simulink model "template_Final_Project_MPC5643L"  (Simulink 7.8)
settings: Solver=FixedStepDiscrete  StartTime=0.0  StopTime=10.0  RelTol=1e-3
InitFcn:
  | parameters
values from neighbouring files (symbols this model uses):
  Ak = 100    [parameters.m]
  b = 100    [parameters.m]
  dT = 0.01    [parameters.m]
  H = 10    [parameters.m]
  Kd_PD = 0.04    [parameters.m]
  Kd_PID = 40    [parameters.m]
  Ki_PID = 0    [parameters.m]
  Kp_PD = 0.4    [parameters.m]
  Kp_PID = 500    [parameters.m]
  L1 = 1.6    [parameters.m]
  L2 = 0.8    [parameters.m]
  m = 2000    [parameters.m]
  V_Ki = 50    [parameters.m]
  V_Kp = 5000    [parameters.m]
undefined symbols (not defined in the file or in its folder): A10, A13, A14, A7, A8, AN0, B, B13, B4, B6, B7, B8, C5, C6, D, D11, D4, DiscIntNeverNeededParam, F15, F3, F4, G4, H4, L3, M14, M3, N15, N3, P3, PA10, PA11, PA12, PA13, PA14, PA5, PA6, PA7, PA8, PA9, PB13, PB7, PC11, PC12, PC13, PC14, PC15, PC6, PD0, PD1, PD10, PD11, PD2, PD3, PD4, PD5, PD6, PD7, PD8, PD9, R10 ... (+4)
libraries: Conv_Lib x54, rappid_564xl_ec_toolbox x50, simulink x19, Veh_Sim x9, U_of_M_5643_blockset x1
(part 1 of 2)
settings Model: Creator=lab  LastModifiedBy=jesseku
settings DataIOCC: ExternalInput=off  InitialState=off  SaveOutput=off  SignalLogging=off  SaveTime=off
settings OptimizationCC: InlineParams=on  OptimizeModelRefInitCode=on  LifeSpan=1
settings DebuggingCC: InheritedTsInSrcMsg=none  SingleTaskRateTransMsg=error  UnconnectedInputMsg=error  UnconnectedOutputMsg=error  UnconnectedLineMsg=error  UnknownTsInhSupMsg=error
settings HardwareCC: ProdLargestAtomicInteger=Long  ProdLargestAtomicFloat=Double  ProdIntDivRoundTo=Zero  ProdEndianess=BigEndian  ProdHWDeviceType=Motorola PowerPC
settings RTWCC: SystemTargetFile=rappid564xl.tlc  MakeCommand=rappid_564xl_make_rtw  TemplateMakefile=rappid_564xl_default_tmf  PostCodeGenCommand=rappid_analyzegencode(buildInfo)  Description=RAppID Toolbox MPC564xL Code Generation Target (rappid)  GenerateReport=on  ProcessScript=rappid564xl_make_rtw_hook  IncludeHyperlinkInReport=on  LaunchReport=on
settings CodeAppCC: IgnoreCustomStorageClasses=off
settings STFCustomTargetCC: GeneratePreprocessorConditionals=Use local settings  CombineOutputUpdateFcns=on  SuppressErrorStatus=on  ERTCustomFileBanners=on  SupportContinuousTime=off  SupportNonInlinedSFcns=off  SystemTargetFile=rappid564xl.tlc
settings ERTTargetCC: MultiwordLength=2048  ParMdlRefBuildCompliant=off  CompOptLevelCompliant=off  ConcurrentExecutionCompliant=off  SuppressErrorStatus=on  ERTFirstTimeCompliant=off  ModelStepFunctionPrototypeControlCompliant=off  CPPClassGenCompliant=off  ExtModeMexFile=noextcomm  InlinedParameterPlacement=NonHierarchical  ERTCustomFileTemplate=example_file_process.tlc  ConvertIfToSwitch=off  SuppressUnreachableDefaultCases=off

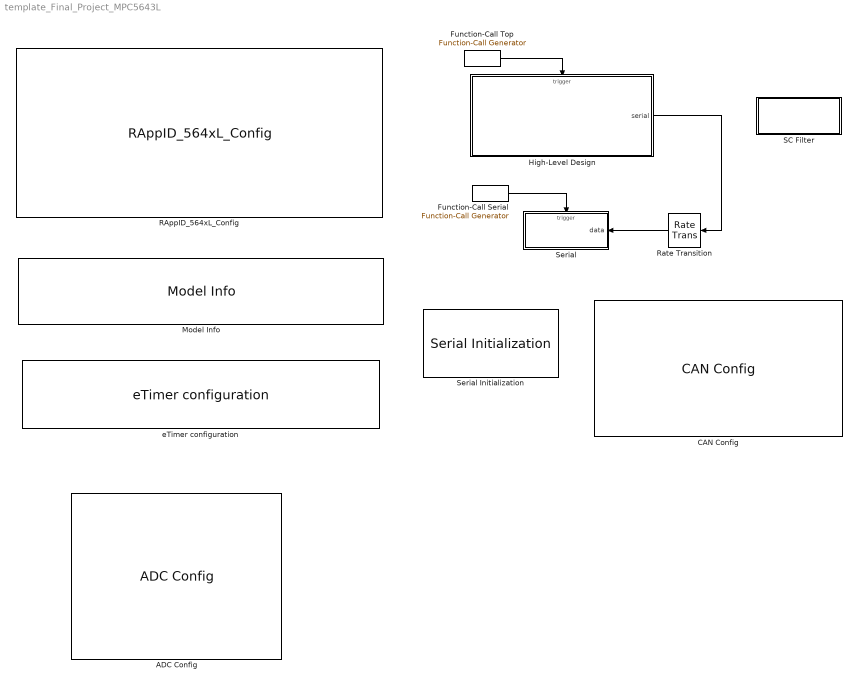
== system template_Final_Project_MPC5643L ==
  ADC Config : rappid_564xl_ec_toolbox/MPC564xL/Motor Control Blocks/ADC Config  adc_unit=0  adc_ctu=off  adc_owr=on  adc_wls=Right  adc_clk=on  adc_ack=on  adc_ctr0_inp=off  adc_ctr0_shft=10 - Avin = 0  adc_ctr0_cmp=01  adc_ctr0_samp=8  adc_ctr1_inp=off  adc_ctr1_cmp=01  adc_ctr1_samp=1  adc_ctr1_tsens=PTAT  adc_pscr_preval=V0  adc_pscr_preconv=off
  CAN Config : rappid_564xl_ec_toolbox/MPC564xL/Communication Blocks/CAN Config  Priority=1  can_unit=A  can_unit_v2=0  can_idam=A - One full ID (standard or extended) per filter element.  can_srx_dis=1 - Self reception disabled  can_presdiv=4  can_rjw=3  can_pseg1=5  can_pseg2=5  can_clk_src=0 - The CAN engine clock source is the oscillator clock  can_lpb=0 - Loop Back disabled  can_smp=0 - One sample is used to determine the bit value  can_boff_rec=0 - Automatic recovering from Bus Off state enabled  can_tsyn=0 - Timer Sync feature disabled  can_lbuf=0 - Buffer with highest priority is transmitted first  can_lom=0 - Listen Only Mode is deactivated  can_propseg=2
  Function-Call Serial : simulink/Ports & Subsystems/Function-Call Generator  sample_time=.05  numberOfIterations=1
  Function-Call Top : simulink/Ports & Subsystems/Function-Call Generator  sample_time=dT  numberOfIterations=1
  High-Level Design : Subsystem
  Model Info : simulink/Model-Wide Utilities/Model Info  InitialBlockCM=None  BlockCM=None  Frame=on  DisplayStringWithTags=|  HorizontalTextAlignment=Center  LeftAlignmentValue=0.5  SourceBlockDiagram=template_Final_Project_MPC5643L  TagMaxNumber=20
      | Model Notes:
      | 
      | You MUST change the CAN IDs whenever you change stations
      | 
      | First 2 buffers must be transmits
  RAppID_564xL_Config : rappid_564xl_ec_toolbox/MPC564xL/RAppID_564xL_Config  SystemClock=120  XTAL=40  MC_clock_60=12  MC_clock_80=16  MC_clock_120=10  SWG_clock_60=20  SWG_clock_80=13.334  SWG_clock_120=20  Compiler=CodeWarrior  MemTarget=FLASH  Part=MPC5643L  Package=144 LQFP  global_int_priority=10  base_tick_priority=11  sys_task_supress=off  exception_handlers=off  stored_mdl_name=adc_pit_block_new  freemaster_interface=Oops  freemaster_rx_pin="LINFlex_0 Rx Pin 116 : \"PB[3]\""  freemaster_tx_pin="LINFlex_0 Tx Pin 114 : \"PB[2]\""  freemaster_interface_1=Serial 0  freemaster_enable=on  freemaster_rate=115200  freemaster_tx0_pin=18 : B[2] : 114 : A14  freemaster_rx0_pin=19 : B[3] : 116 : B13  freemaster_tx1_pin=57 : D[9] : 26 : L3  freemaster_rx1_pin=29 : B[13] : 60 : R10  freemaster_can_channel=1CH  freemater_can_speed=500K  freemaster_can_msgig=0x7AA  ccp_interface=None  ccp_enable=off  ccp_can_channel=CH1 (MB 0 - 1)  ccp_can_speed=500K  ccp_can_cro_id=256  ccp_can_dto_id=257  ccp_dev_id=RappID  ccp_dev_addr=0  ccp_odt=3  ccp_daq=3  pil_enable=off  pil_bam=off  comport=4  pil_rate=115200  bam_password_def=on  bam_password=0xFEEDFACECAFEBEEF  bam_sa_cs=off  bam_start_address=0x0  bam_code_size=0x7000  cons_dspi=on  cons_can=on  cons_adc=on  cons_pwm=on  cons_ctu=on  cons_swg=on  cons_eTimer=on  cons_fm=on
  Rate Transition : RateTransition
  SC Filter : Subsystem
  Serial : Subsystem
  Serial Initialization : U_of_M_5643_blockset/Serial/Serial Initialization
  eTimer configuration : rappid_564xl_ec_toolbox/MPC564xL/Motor Control Blocks/eTimer configuration  SubModule=0  TimerChan=0  subMod=0  channel=0  CountMode=100 - Quadrature count mode using primary and secondary sources  CNTMODE=4  CountOnce=0 - Count repeatedly  ONCE=0  CountLength=0 - Continue counting to roll over  LENGTH=0  CountDirection=0 - Count up  DIR=0  OutputEnable=0 - The external pin is configured as an input  OEN=0  CoChanInit=00 - Other channels cannot force re-initialization of this channel  COINIT=0  StopAction=0 - Output enable is unaffected by stop mode  STPEN=0  ReloadOnCapt=00 - Do not reload the counter on a capture event  ROC=0  PrimarySource=00000 - Counter #0 input pin  PRISRC=0  PrimSrcPol=0 - True polarity  PIPS=0  SecondarySource=00001 - Counter #1 input pin  SECSRC=1  SecSrcPol=0 - True polarity  SIPS=0  FILT_CNT=0  FILT_PER=0  FILT=0  OutputMode=0000 - Software controlled  OUTMODE=0  OutputPol=0 - True polarity  OPS=0  MasterMode=0 - Disable broadcast of this channel output  MSTR=0  ForcedOutVal=0  VAL=0  CoForce=0 - Other channels cannot force this channel output  COFRC=0  CompLoad1=000 - COMP1 is never preload  CLC1=0  CompLoad2=000 - COMP2 is never preload  CLC2=0  CompareMode="00 - COMP1 and COMP2  are used when the counter is counting up"  CMPMODE=0  CaptMode1=00 - Capture disabled  CPT1MODE=0  CaptMode2=00 - Capture disabled  CPT2MODE=0  OneShCaptMode=0 - Free running mode is selected  ONESHOT=0  CaptFIFO=0  CFWM=0  CNTRinit=0  COMP1init=0  COMP2init=0  mod0ch0pin="0   : PA0  : [ 73 ] : [ T14 ]  input/output"  mod0ch1pin="1   : PA1  : [ 74 ] : [ R14 ]  input/output"  mod0ch2pin=None  mod0ch3pin=None  mod0ch4pin=None  mod0ch5pin=None  mod1ch0pin=None  mod1ch1pin=None  mod1ch2pin=None  mod1ch3pin=None  mod1ch4pin=None  mod1ch5pin=None  mod2ch0pin=None  mod2ch1pin=None  mod2ch2pin=None  mod2ch3pin=None  mod2ch4pin=None  mod2ch5pin=None  pcrNum0=0  pcrNum1=1  pcrNum2=255  pcrNum3=255  pcrNum4=255  pcrNum5=255  TCFIE=off  TCF1IE=off  TCF2IE=off  TOFIE=off  IELFIE=off  IEHFIE=off  ICF1IE=off  ICF2IE=off  INTDMA=0
  wires:
  Function-Call Serial/1 -> Serial/Trigger
  Rate Transition/1 -> Serial/1(data)
  Function-Call Top/1 -> High-Level Design/Trigger
  High-Level Design/1(serial) -> Rate Transition/1

== system template_Final_Project_MPC5643L/High-Level Design ==
  Trigger : TriggerPort  TriggerType=function-call
  ACC : Subsystem
  Inputs : Subsystem
  Outputs : Subsystem
  Vehicle_Model : Subsystem
  serial : Outport
  wires:
  Outputs/1(x,y,psi (Cars 1 - 6)) -> serial/1
  Inputs/2(ACC_enable) -> ACC/1(ACC_enable)
  Inputs/1(s,n,psi,us (Cars 1 - 6)) -> ACC/2(s.n.psi,us (Cars 1-6)), Outputs/1(s,n,psi,us (Cars 1 - 6))
  Inputs/3(Cruise Control Speed) -> ACC/3(Cruise Control Speed)
  Inputs/4(Steering Angle (delta)) -> ACC/4(delta)
  Inputs/6(Automatic Steering_enable) -> ACC/6(Automatic Steering_enable)
  ACC/1(Force) -> Vehicle_Model/1(Fd)
  ACC/2(delta (out)) -> Vehicle_Model/2(delta)
  ACC/3(self-aligning torque (out)) -> Vehicle_Model/3(self-align torque (in))
  ACC/4(auto torque (out)) -> Vehicle_Model/4(auto torque (in))
  Vehicle_Model/2(u) -> Outputs/3(u (This Car)), ACC/8(u (in))
  Vehicle_Model/3(self-aligning torque) -> Outputs/4(Self-aligning torque)
  Vehicle_Model/4(auto torque) -> Outputs/5(Auto torque)
  Vehicle_Model/1(s,n,psi,us) -> Outputs/2(s,n,psi,us (This Car)), ACC/7(s.n.psi,us (This Car))
  Inputs/5(Throttle (Fd)) -> ACC/5(Fd)

== system template_Final_Project_MPC5643L/SC Filter ==
  Constant1 : Constant  Value=1e6  OutDataTypeStr=uint32
  Constant2 : Constant  Value=0  OutDataTypeStr=uint32
  Constant3 : Constant  Value=50  OutDataTypeStr=uint32
  Simple PWM Output : rappid_564xl_ec_toolbox/MPC564xL/Motor Control Blocks/Simple PWM Output  Priority=1  pwmModule=0  pwmMod=0  SubModule=1  subMod=1  InitFreq=1000000  resolution=1 %  resValue=1  InitDutyA=0  InitDutyB=50  align=A B - edge aligned  PhaseShift_A=0  PhaseShift=0  Phase_A=0  Phase_B=0  centered=0  DoubleS=off  doubleSw=off  debugSw=off  debug_mode=0  pin_A0=None  pin_B0=None  pin_X0=None  pin_A1=None  pin_B1="38  : PC6  : [ 142 ] : [ D4 ]"  pin_X1=None  pin_A2=None  pin_B2=None  pin_X2=None  pin_A3=None  pin_B3=None  pin_X3=None  pin1_A0=None  pin1_B0=None  pin1_X0=None  pin1_A1=None  pin1_B1=None  pin1_X1=None  pin1_A2=None  pin1_B2=None  pin1_X2=None  pin1_A3=None  pin1_B3=None  pin1_X3=None  pcrNumA=255  pcrNumB=38  pcrNumX=255  polA=off  polB=off  polX=off  octrl=0  syncFrom0=off  masterSync=0  outVal0=off  outVal1=off  outVal2=off  outVal3=off  outVal4=on  outVal5=on  outTrig=48
  wires:
  Constant1/1 -> Simple PWM Output/1
  Constant2/1 -> Simple PWM Output/2
  Constant3/1 -> Simple PWM Output/3

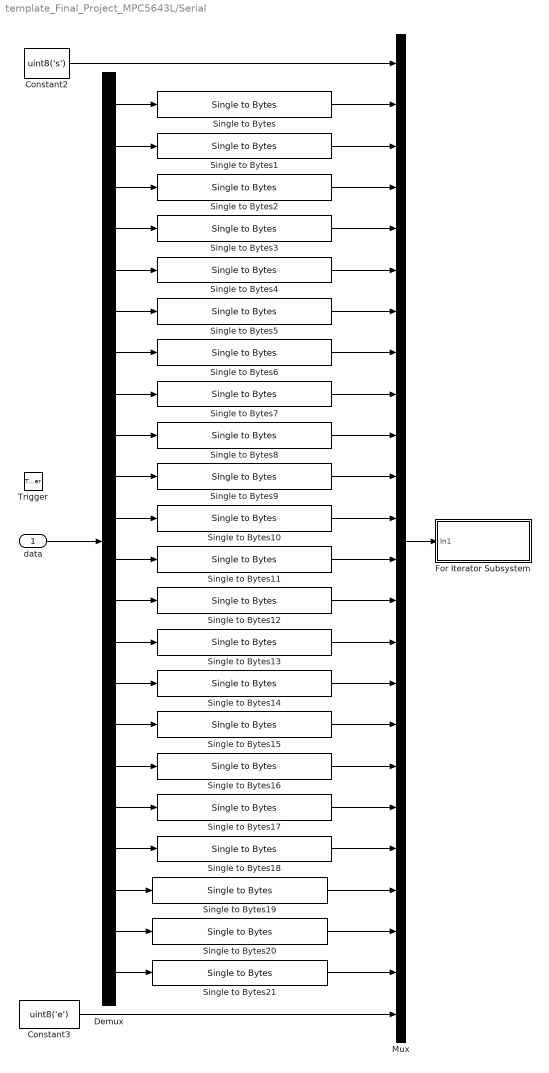
== system template_Final_Project_MPC5643L/Serial ==
  data : Inport
  Trigger : TriggerPort  TriggerType=function-call
  Constant2 : Constant  Value=uint8('s')  OutDataTypeStr=uint8
  Constant3 : Constant  Value=uint8('e')  OutDataTypeStr=uint8
  Demux : Demux  Outputs=22
  For Iterator Subsystem : Subsystem
  Mux : Mux  Inputs=24
  Single to Bytes{,1..21} (22 alike) : Conv_Lib/Single to Bytes
  wires:
  Constant2/1 -> Mux/1
  Single to Bytes/1 -> Mux/2
  Single to Bytes1/1 -> Mux/3
  Single to Bytes2/1 -> Mux/4
  Single to Bytes3/1 -> Mux/5
  Single to Bytes4/1 -> Mux/6
  Single to Bytes5/1 -> Mux/7
  Single to Bytes6/1 -> Mux/8
  Single to Bytes7/1 -> Mux/9
  Single to Bytes8/1 -> Mux/10
  Single to Bytes9/1 -> Mux/11
  Single to Bytes10/1 -> Mux/12
  Single to Bytes11/1 -> Mux/13
  Single to Bytes12/1 -> Mux/14
  Single to Bytes13/1 -> Mux/15
  Single to Bytes15/1 -> Mux/17
  Single to Bytes16/1 -> Mux/18
  Single to Bytes17/1 -> Mux/19
  Mux/1 -> For Iterator Subsystem/1(In1)
  Demux/1 -> Single to Bytes/1
  Demux/2 -> Single to Bytes1/1
  Demux/3 -> Single to Bytes2/1
  Demux/4 -> Single to Bytes3/1
  Demux/5 -> Single to Bytes4/1
  Demux/6 -> Single to Bytes5/1
  Demux/7 -> Single to Bytes6/1
  Demux/8 -> Single to Bytes7/1
  Demux/9 -> Single to Bytes8/1
  Demux/10 -> Single to Bytes9/1
  Demux/11 -> Single to Bytes10/1
  Demux/12 -> Single to Bytes11/1
  Demux/13 -> Single to Bytes12/1
  Demux/14 -> Single to Bytes13/1
  Demux/15 -> Single to Bytes14/1
  Demux/16 -> Single to Bytes15/1
  Demux/17 -> Single to Bytes16/1
  Demux/18 -> Single to Bytes17/1
  data/1 -> Demux/1
  Single to Bytes14/1 -> Mux/16
  Demux/19 -> Single to Bytes18/1
  Demux/20 -> Single to Bytes19/1
  Demux/21 -> Single to Bytes20/1
  Demux/22 -> Single to Bytes21/1
  Single to Bytes18/1 -> Mux/20
  Single to Bytes19/1 -> Mux/21
  Single to Bytes20/1 -> Mux/22
  Single to Bytes21/1 -> Mux/23
  Constant3/1 -> Mux/24

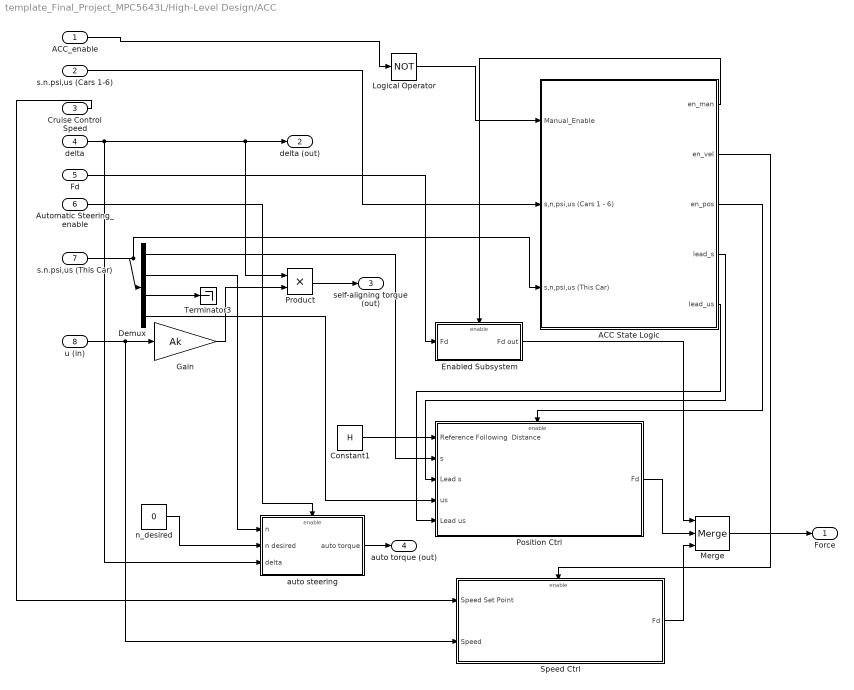
== system template_Final_Project_MPC5643L/High-Level Design/ACC ==
  ACC_enable : Inport
  s.n.psi,us (Cars 1-6) : Inport  Port=2
  Cruise Control Speed : Inport  Port=3
  delta : Inport  Port=4
  Fd : Inport  Port=5
  Automatic Steering_enable : Inport  Port=6
  s.n.psi,us (This Car) : Inport  Port=7
  u (in) : Inport  Port=8
  ACC State Logic : Subsystem
  Constant1 : Constant  Value=H  OutDataTypeStr=single
  Demux : Demux
  Enabled Subsystem : Subsystem  TreatAsAtomicUnit=on
  Gain : Gain  Gain=Ak
  Logical Operator : Logic  Operator=NOT  AllPortsSameDT=off  OutDataTypeStr=boolean
  Merge : Merge  Inputs=3
  Position Ctrl : Subsystem  TreatAsAtomicUnit=on
  Product : Product  OutDataTypeStr=single  RndMeth=Zero
  Speed Ctrl : Subsystem  TreatAsAtomicUnit=on
  Terminator3 : Terminator
  auto steering : Subsystem  TreatAsAtomicUnit=on
  n_desired : Constant  Value=0  OutDataTypeStr=single
  Force : Outport  OutDataTypeStr=single
  delta (out) : Outport  Port=2
  self-aligning torque (out) : Outport  Port=3
  auto torque (out) : Outport  Port=4
  wires:
  ACC_enable/1 -> Logical Operator/1
  delta/1 -> auto steering/3(delta), Product/1, delta (out)/1
  u (in)/1 -> Gain/1, Speed Ctrl/2(Speed)
  Gain/1 -> Product/2
  Product/1 -> self-aligning torque (out)/1
  Logical Operator/1 -> ACC State Logic/1(Manual_Enable)
  s.n.psi,us (Cars 1-6)/1 -> ACC State Logic/2(s,n,psi,us (Cars 1 - 6))
  ACC State Logic/3(en_pos) -> Position Ctrl/Enable
  ACC State Logic/2(en_vel) -> Speed Ctrl/Enable
  ACC State Logic/4(lead_s) -> Position Ctrl/3(Lead s)
  ACC State Logic/5(lead_us) -> Position Ctrl/5(Lead us)
  Cruise Control Speed/1 -> Speed Ctrl/1(Speed Set Point)
  s.n.psi,us (This Car)/1 -> ACC State Logic/3(s,n,psi,us (This Car)), Demux/1
  Demux/1 -> Position Ctrl/2(s)
  Demux/4 -> Position Ctrl/4(us)
  Demux/3 -> Terminator3/1
  Constant1/1 -> Position Ctrl/1(Reference Following  Distance)
  Position Ctrl/1(Fd) -> Merge/2
  Speed Ctrl/1(Fd) -> Merge/3
  Merge/1 -> Force/1
  ACC State Logic/1(en_man) -> Enabled Subsystem/Enable
  Enabled Subsystem/1(Fd out) -> Merge/1
  Fd/1 -> Enabled Subsystem/1(Fd)
  auto steering/1(auto torque) -> auto torque (out)/1
  Demux/2 -> auto steering/1(n)
  n_desired/1 -> auto steering/2(n desired)
  Automatic Steering_enable/1 -> auto steering/Enable

== system template_Final_Project_MPC5643L/High-Level Design/Inputs ==
  ADC Channel : rappid_564xl_ec_toolbox/MPC564xL/Motor Control Blocks/ADC Channel  adc_unit=0  adc_chan0=older  adc_chan0_v2=23 : PB7 : [43] : [R5] : AN0  adc_chan1=older  adc_chan1_v2=29 : PB13 : [60] : [R10] : AN0  simulate=off  interrupt=off  adc_mode=Normal  adc_presample=off
  Data Type Conversion : DataTypeConversion  OutDataTypeStr=single
  Digital Input : rappid_564xl_ec_toolbox/MPC564xL/General Purpose Blocks/Digital Input  gpio_outputs="13  : PA13 : [ 136 ] : [ C6 ]"  pinNum=[ 136 ]  pcrNum=13
  Digital Input1 : rappid_564xl_ec_toolbox/MPC564xL/General Purpose Blocks/Digital Input  gpio_outputs="14  : PA14 : [ 143 ] : [ B4 ]"  pinNum=[ 143 ]  pcrNum=14
  Other Cars : Subsystem
  Scale1 : Subsystem
  Speed_input : Subsystem
  eTimer CNTR Register Read : rappid_564xl_ec_toolbox/MPC564xL/Motor Control Blocks/eTimer CNTR Register Read  SubModule=0  TimerChan=0  subMod=0  channel=0
  s,n,psi,us (Cars 1 - 6) : Outport
  ACC_enable : Outport  Port=2
  Cruise Control Speed : Outport  Port=3
  Steering Angle (delta) : Outport  Port=4
  Throttle (Fd) : Outport  Port=5
  Automatic Steering_enable : Outport  Port=6
  wires:
  Digital Input1/1 -> Automatic Steering_enable/1
  Other Cars/1(s,n,psi,us (Car 1 - 6)) -> s,n,psi,us (Cars 1 - 6)/1
  Digital Input/1 -> ACC_enable/1
  eTimer CNTR Register Read/1 -> Scale1/1(Encoder Counts)
  Scale1/1(Haptic Wheel Position (degrees)) -> Steering Angle (delta)/1
  Speed_input/1(Command Speed) -> Cruise Control Speed/1
  ADC Channel/1 -> Data Type Conversion/1
  Data Type Conversion/1 -> Throttle (Fd)/1

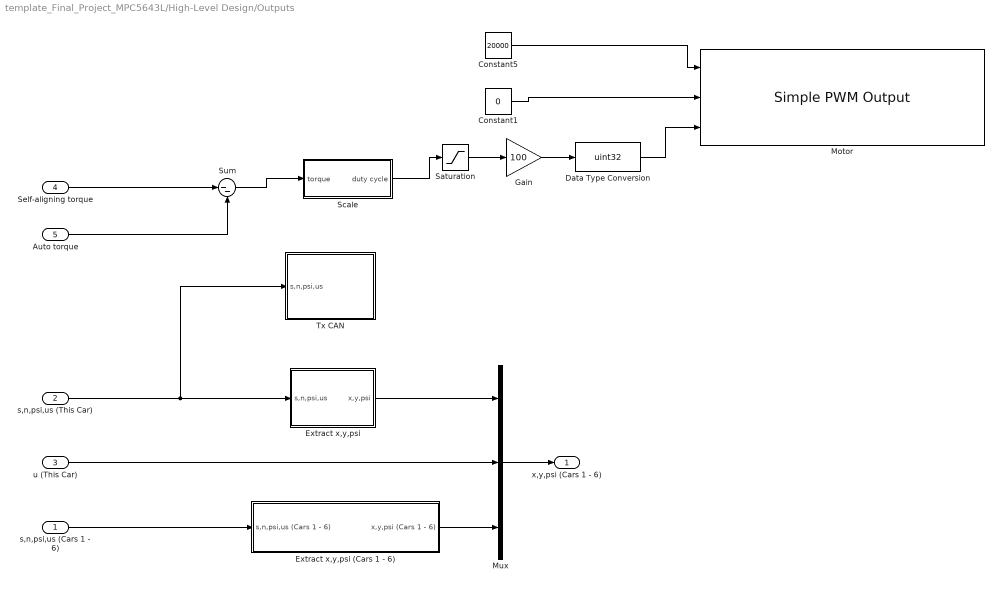
== system template_Final_Project_MPC5643L/High-Level Design/Outputs ==
  s,n,psi,us (Cars 1 - 6) : Inport
  s,n,psi,us (This Car) : Inport  Port=2
  u (This Car) : Inport  Port=3
  Self-aligning torque : Inport  Port=4
  Auto torque : Inport  Port=5
  Constant1 : Constant  Value=0  OutDataTypeStr=uint32
  Constant5 : Constant  Value=20000  OutDataTypeStr=uint32
  Data Type Conversion : DataTypeConversion  OutDataTypeStr=uint32
  Extract x,y,psi : Subsystem
  Extract x,y,psi (Cars 1 - 6) : Subsystem
  Gain : Gain  Gain=100
  Motor : rappid_564xl_ec_toolbox/MPC564xL/Motor Control Blocks/Simple PWM Output  Priority=1  pwmModule=0  pwmMod=0  SubModule=0  subMod=0  InitFreq=20000  resolution=1 %  resValue=1  InitDutyA=0  InitDutyB=0  align=A B - edge aligned  PhaseShift_A=0  PhaseShift=0  Phase_A=0  Phase_B=0  centered=0  DoubleS=off  doubleSw=off  debugSw=off  debug_mode=0  pin_A0=None  pin_B0="59  : PD11 : [ 78 ] : [ R16 ]"  pin_X0=None  pin_A1=None  pin_B1=None  pin_X1=None  pin_A2=None  pin_B2=None  pin_X2=None  pin_A3=None  pin_B3=None  pin_X3=None  pin1_A0=None  pin1_B0=None  pin1_X0=None  pin1_A1=None  pin1_B1=None  pin1_X1=None  pin1_A2=None  pin1_B2=None  pin1_X2=None  pin1_A3=None  pin1_B3=None  pin1_X3=None  pcrNumA=255  pcrNumB=59  pcrNumX=255  polA=off  polB=off  polX=off  octrl=0  syncFrom0=off  masterSync=0  outVal0=off  outVal1=off  outVal2=on  outVal3=on  outVal4=on  outVal5=on  outTrig=60
  Mux : Mux  Inputs=3
  Saturation : Saturate  UpperLimit=.76  LowerLimit=.24
  Scale : Subsystem
  Sum : Sum  Inputs=|--
  Tx CAN : Subsystem
  x,y,psi (Cars 1 - 6) : Outport
  wires:
  s,n,psi,us (Cars 1 - 6)/1 -> Extract x,y,psi (Cars 1 - 6)/1(s,n,psi,us (Cars 1 - 6))
  s,n,psi,us (This Car)/1 -> Extract x,y,psi/1(s,n,psi,us), Tx CAN/1(s,n,psi,us)
  Extract x,y,psi/1(x,y,psi) -> Mux/1
  Mux/1 -> x,y,psi (Cars 1 - 6)/1
  u (This Car)/1 -> Mux/2
  Extract x,y,psi (Cars 1 - 6)/1(x,y,psi (Cars 1 - 6)) -> Mux/3
  Constant1/1 -> Motor/2
  Constant5/1 -> Motor/1
  Saturation/1 -> Gain/1
  Scale/1(duty cycle) -> Saturation/1
  Gain/1 -> Data Type Conversion/1
  Data Type Conversion/1 -> Motor/3
  Sum/1 -> Scale/1(torque)
  Self-aligning torque/1 -> Sum/1
  Auto torque/1 -> Sum/2

== system template_Final_Project_MPC5643L/High-Level Design/Vehicle_Model ==
  Fd : Inport  OutDataTypeStr=single
  delta : Inport  Port=2  OutDataTypeStr=single
  self-align torque (in) : Inport  Port=3
  auto torque (in) : Inport  Port=4
  DTC1 : DataTypeConversion  OutDataTypeStr=single
  DTC2 : DataTypeConversion  OutDataTypeStr=single
  Mux : Mux
  Subsystem : Subsystem
  u to us : Subsystem
  x,y to s,n : Veh_Sim/x,y to s,n  SystemSampleTime=-1
  s,n,psi,us : Outport
  u : Outport  Port=2
  self-aligning torque : Outport  Port=3
  auto torque : Outport  Port=4
  wires:
  Fd/1 -> DTC1/1
  delta/1 -> DTC2/1
  DTC1/1 -> Subsystem/1(Fd)  "Fd"
  DTC2/1 -> u to us/3(delta), Subsystem/2(delta)  "delta"
  self-align torque (in)/1 -> self-aligning torque/1
  auto torque (in)/1 -> auto torque/1
  Subsystem/1(x) -> x,y to s,n/1
  Subsystem/2(y) -> x,y to s,n/2
  Subsystem/4(u) -> u/1, u to us/4(u)
  Subsystem/3(psi) -> u to us/2(psi), Mux/3
  x,y to s,n/1 -> u to us/1(s), Mux/1
  x,y to s,n/2 -> Mux/2
  Mux/1 -> s,n,psi,us/1
  u to us/1(us) -> Mux/4

== system template_Final_Project_MPC5643L/Serial/For Iterator Subsystem ==
  In1 : Inport
  Data Type Conversion : DataTypeConversion  OutDataTypeStr=uint8
  For Iterator : ForIterator  IterationLimit=91  IndexMode=Zero-based  IterationVariableDataType=int8
  Index Vector : MultiPortSwitch  DataPortOrder=Zero-based contiguous  Inputs=1  zeroidx=on
  S-Function : S-Function  FunctionName=SerialSend  EnableBusSupport=off
      mask Display:
      | patch([0 0 1 1], [0 1 1 0], [255/255 255/255 0])
      | patch([0 0 0.05 0.05], [0 1 1 0], [0 0 255/255])
      | patch([1 1 0.95 0.95], [0 1 1 0], [0 0 255/255])
      | 
      | text (0.52, 0.8, ['Serial Send'], 'horizontalAlignment', 'center');
      | %text (0.5, .5, ['System Clock MHz: ' get_param(gcb,'SystemClock')], 'horizontalAlignment', 'center');
      | %text (0.5, .35, ['Baud Rate: ' get_param(gcb,'BaudRate')], 'horizontalAlignment', 'center');
      | text(0.5, 0.1, 'The University of Michigan', 'horizontalAlignment', 'center');
  wires:
  In1/1 -> Index Vector/2
  Index Vector/1 -> Data Type Conversion/1
  For Iterator/1 -> Index Vector/1
  Data Type Conversion/1 -> S-Function/1

== system template_Final_Project_MPC5643L/High-Level Design/ACC/ACC State Logic ==
  Manual_Enable : Inport
  s,n,psi,us (Cars 1 - 6) : Inport  Port=2
  s,n,psi,us (This Car) : Inport  Port=3
  Chart : Stateflow chart  TreatAsAtomicUnit=on
  Constant : Constant  Value=H  OutDataTypeStr=single
  Demux1 : Demux
  Pick_Lead : Subsystem
  Terminator : Terminator
  Terminator16 : Terminator
  Terminator17 : Terminator
  en_man : Outport
  en_vel : Outport  Port=2
  en_pos : Outport  Port=3
  lead_s : Outport  Port=4
  lead_us : Outport  Port=5
  wires:
  Demux1/1 -> Pick_Lead/3(s), Chart/5(s)
  Demux1/2 -> Terminator16/1
  Demux1/3 -> Terminator17/1
  Demux1/4 -> Chart/4(us)
  s,n,psi,us (Cars 1 - 6)/1 -> Pick_Lead/2(si)
  Constant/1 -> Pick_Lead/1(H), Chart/6(H)
  s,n,psi,us (This Car)/1 -> Demux1/1
  Pick_Lead/1(lead_s) -> lead_s/1, Chart/3(si)
  Pick_Lead/2(lead_u) -> lead_us/1, Chart/2(usi)
  Manual_Enable/1 -> Chart/1(enable)
  Chart/1(speed_en) -> en_vel/1
  Chart/2(pos_en) -> en_pos/1
  Chart/3(man_en) -> en_man/1
  Chart/4(state) -> Terminator/1

== system template_Final_Project_MPC5643L/High-Level Design/ACC/Enabled Subsystem ==
  Fd : Inport  OutDataTypeStr=single
  Enable : EnablePort
  Fd out : Outport  OutDataTypeStr=single
  wires:
  Fd/1 -> Fd out/1

== system template_Final_Project_MPC5643L/High-Level Design/ACC/Position Ctrl ==
  note: u
  Reference Following  Distance : Inport
  s : Inport  Port=2
  Lead s : Inport  Port=3
  us : Inport  Port=4
  Lead us : Inport  Port=5
  Enable : EnablePort
  D-gain : Gain  Gain=2.45*m  SaturateOnIntegerOverflow=on  OutDataTypeStr=Inherit: Same as input  ParamDataTypeStr=Inherit: Same as input
  Feed-forward : Gain  Gain=b  SaturateOnIntegerOverflow=on  OutDataTypeStr=Inherit: Same as input  ParamDataTypeStr=Inherit: Same as input
  P-gain : Gain  Gain=-1.5*m  SaturateOnIntegerOverflow=on  OutDataTypeStr=Inherit: Same as input  ParamDataTypeStr=Inherit: Same as input
  Sum1 : Sum  Inputs=|++  SaturateOnIntegerOverflow=on
  Sum2 : Sum  Inputs=+-|  SaturateOnIntegerOverflow=on
  Sum3 : Sum  Inputs=|+-  SaturateOnIntegerOverflow=on
  Sum4 : Sum  Inputs=|+-  SaturateOnIntegerOverflow=on
  Sum5 : Sum  Inputs=|++  SaturateOnIntegerOverflow=on
  Fd : Outport
  wires:
  Lead s/1 -> Sum3/1
  s/1 -> Sum3/2
  Reference Following  Distance/1 -> Sum2/1  "desired distance"
  Sum3/1 -> Sum2/2  "head-way"
  Sum2/1 -> P-gain/1
  P-gain/1 -> Sum1/1
  D-gain/1 -> Sum1/2
  us/1 -> Sum4/2
  Lead us/1 -> Sum4/1, Feed-forward/1
  Sum4/1 -> D-gain/1
  Feed-forward/1 -> Sum5/2
  Sum1/1 -> Sum5/1
  Sum5/1 -> Fd/1  "F"

== system template_Final_Project_MPC5643L/High-Level Design/ACC/Speed Ctrl ==
  Speed Set Point : Inport
  Speed : Inport  Port=2
  Enable : EnablePort
  Gain : Gain  Gain=b  SaturateOnIntegerOverflow=on  OutDataTypeStr=Inherit: Same as input  ParamDataTypeStr=Inherit: Same as input
  PI : Subsystem
  Sum : Sum  Inputs=++|  SaturateOnIntegerOverflow=on
  Sum1 : Sum  Inputs=|+-  SaturateOnIntegerOverflow=on
  Fd : Outport
  wires:
  Speed Set Point/1 -> Gain/1, Sum1/1  "desired speed"
  Speed/1 -> Sum1/2
  Sum1/1 -> PI/1(Error)
  Gain/1 -> Sum/1
  PI/1(U) -> Sum/2
  Sum/1 -> Fd/1  "Fd"

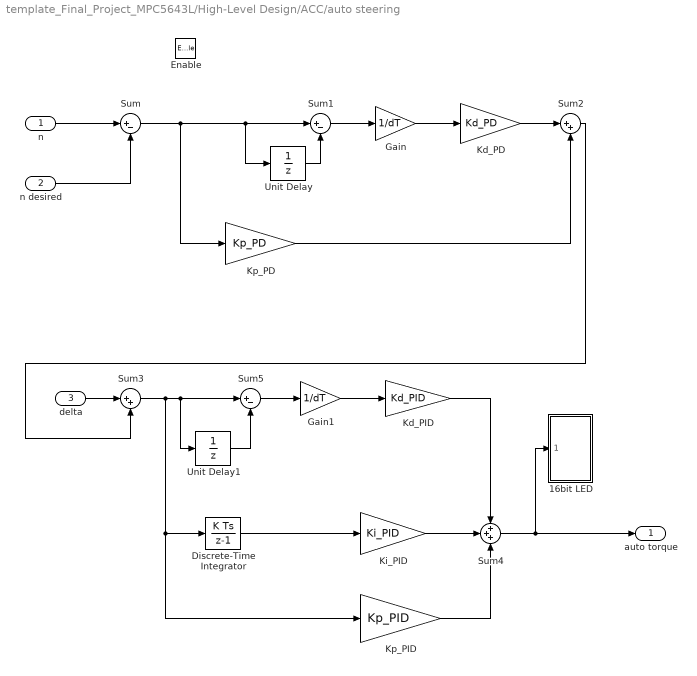
== system template_Final_Project_MPC5643L/High-Level Design/ACC/auto steering ==
  n : Inport
  n desired : Inport  Port=2
  delta : Inport  Port=3
  Enable : EnablePort
  16bit LED : Subsystem
  Discrete-Time Integrator : DiscreteIntegrator  SampleTime=-1  ICPrevOutput=DiscIntNeverNeededParam  ICPrevScaledInput=DiscIntNeverNeededParam
  Gain : Gain  Gain=1/dT
  Gain1 : Gain  Gain=1/dT
  Kd_PD : Gain  Gain=Kd_PD
  Kd_PID : Gain  Gain=Kd_PID
  Ki_PID : Gain  Gain=Ki_PID
  Kp_PD : Gain  Gain=Kp_PD
  Kp_PID : Gain  Gain=Kp_PID
  Sum : Sum  Inputs=|+-
  Sum1 : Sum  Inputs=|+-
  Sum2 : Sum  Inputs=|++
  Sum3 : Sum  Inputs=|++
  Sum4 : Sum  Inputs=+++
  Sum5 : Sum  Inputs=|+-
  Unit Delay : UnitDelay  SampleTime=-1
  Unit Delay1 : UnitDelay  SampleTime=-1
  auto torque : Outport
  wires:
  n/1 -> Sum/1
  n desired/1 -> Sum/2
  Sum/1 -> Sum1/1, Unit Delay/1, Kp_PD/1
  Unit Delay/1 -> Sum1/2
  Sum1/1 -> Gain/1
  Gain/1 -> Kd_PD/1
  Kd_PD/1 -> Sum2/1
  Kp_PD/1 -> Sum2/2
  delta/1 -> Sum3/1
  Kd_PID/1 -> Sum4/1
  Ki_PID/1 -> Sum4/2
  Kp_PID/1 -> Sum4/3
  Discrete-Time Integrator/1 -> Ki_PID/1
  Sum3/1 -> Kp_PID/1, Discrete-Time Integrator/1, Sum5/1, Unit Delay1/1
  Gain1/1 -> Kd_PID/1
  Sum5/1 -> Gain1/1
  Unit Delay1/1 -> Sum5/2
  Sum4/1 -> 16bit LED/1(16 bits), auto torque/1
  Sum2/1 -> Sum3/2

== system template_Final_Project_MPC5643L/High-Level Design/Inputs/Other Cars ==
  "1 for GSI vehicle only, 0 for ALL student vehicles" : Constant  Value=0
  Car1 : Subsystem
  Car2 : Subsystem
  Car3 : Subsystem
  Car4 : Subsystem
  Car5 : Subsystem
  Car6 : Subsystem
  GSI Car : Subsystem
  Mux1 : Mux  Inputs=2
  Mux2 : Mux  Inputs=6
  Switch : Switch  Criteria=u2 ~= 0
  Zeros (20) : Subsystem
  s,n,psi,us (Car 1 - 6) : Outport
  wires:
  GSI Car/1(s,n,psi,us) -> Mux1/1
  Zeros (20)/1(Zeros) -> Mux1/2
  Mux1/1 -> Switch/1
  Switch/1 -> s,n,psi,us (Car 1 - 6)/1
  "1 for GSI vehicle only, 0 for ALL student vehicles"/1 -> Switch/2
  Car1/1(s,n,psi,us) -> Mux2/1
  Car2/1(s,n,psi,us) -> Mux2/2
  Car3/1(s,n,psi,us) -> Mux2/3
  Car4/1(s,n,psi,us) -> Mux2/4
  Car5/1(s,n,psi,us) -> Mux2/5
  Mux2/1 -> Switch/3
  Car6/1(s,n,psi,us) -> Mux2/6

== system template_Final_Project_MPC5643L/High-Level Design/Inputs/Scale1 ==
  Encoder Counts : Inport
  Data Type Conversion : DataTypeConversion  OutDataTypeStr=uint16
  Data Type Conversion1 : DataTypeConversion  OutDataTypeStr=int16
  Data Type Conversion2 : DataTypeConversion  OutDataTypeStr=single
  Gain : Gain  Gain=.09
  Gain1 : Gain  Gain=pi/1800
  Sum : Sum  Inputs=|+-
  Sum1 : Sum  Inputs=|++
  Unit Delay : UnitDelay  SampleTime=-1
  Unit Delay1 : UnitDelay  SampleTime=-1
  Haptic Wheel Position (degrees) : Outport
  wires:
  Encoder Counts/1 -> Data Type Conversion/1
  Data Type Conversion/1 -> Unit Delay/1, Sum/1
  Unit Delay/1 -> Sum/2
  Sum/1 -> Data Type Conversion1/1
  Data Type Conversion1/1 -> Data Type Conversion2/1
  Data Type Conversion2/1 -> Gain/1
  Sum1/1 -> Unit Delay1/1, Gain1/1
  Unit Delay1/1 -> Sum1/2
  Gain/1 -> Sum1/1
  Gain1/1 -> Haptic Wheel Position (degrees)/1

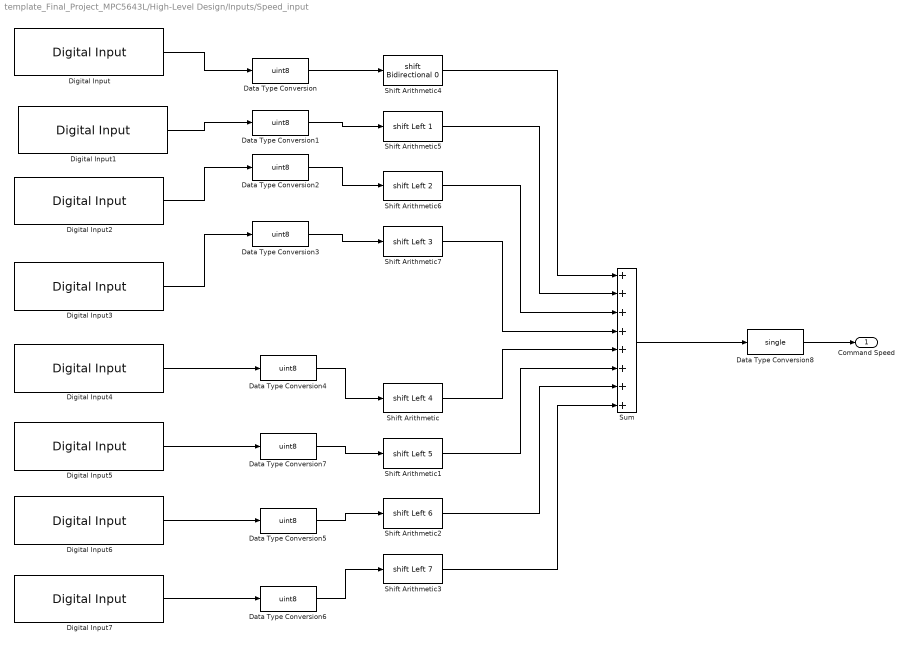
== system template_Final_Project_MPC5643L/High-Level Design/Inputs/Speed_input ==
  Data Type Conversion{,1..7} (8 alike) : DataTypeConversion  OutDataTypeStr=uint8
  Data Type Conversion8 : DataTypeConversion  OutDataTypeStr=single
  Digital Input : rappid_564xl_ec_toolbox/MPC564xL/General Purpose Blocks/Digital Input  gpio_outputs="5   : PA5  : [ 14 ] : [ H4 ]"  pinNum=[ 14 ]  pcrNum=5
  Digital Input1 : rappid_564xl_ec_toolbox/MPC564xL/General Purpose Blocks/Digital Input  gpio_outputs="6   : PA6  : [ 2 ] : [ G4 ]"  pinNum=[ 2 ]  pcrNum=6
  Digital Input2 : rappid_564xl_ec_toolbox/MPC564xL/General Purpose Blocks/Digital Input  gpio_outputs="7   : PA7  : [ 10 ] : [ F3 ]"  pinNum=[ 10 ]  pcrNum=7
  Digital Input3 : rappid_564xl_ec_toolbox/MPC564xL/General Purpose Blocks/Digital Input  gpio_outputs="8   : PA8  : [ 12 ] : [ F4 ]"  pinNum=[ 12 ]  pcrNum=8
  Digital Input4 : rappid_564xl_ec_toolbox/MPC564xL/General Purpose Blocks/Digital Input  gpio_outputs="9   : PA9  : [ 134 ] : [ B6 ]"  pinNum=[ 134 ]  pcrNum=9
  Digital Input5 : rappid_564xl_ec_toolbox/MPC564xL/General Purpose Blocks/Digital Input  gpio_outputs="10  : PA10  : [ 118 ] : [ A13 ]"  pinNum=[ 118 ]  pcrNum=10
  Digital Input6 : rappid_564xl_ec_toolbox/MPC564xL/General Purpose Blocks/Digital Input  gpio_outputs="11  : PA11 : [ 120 ] : [ D11 ]"  pinNum=[ 120 ]  pcrNum=11
  Digital Input7 : rappid_564xl_ec_toolbox/MPC564xL/General Purpose Blocks/Digital Input  gpio_outputs="12  : PA12 : [ 122 ] : [ A10 ]"  pinNum=[ 122 ]  pcrNum=12
  Shift Arithmetic : ArithShift  BitShiftNumber=4  BitShiftDirection=Left
  Shift Arithmetic1 : ArithShift  BitShiftNumber=5  BitShiftDirection=Left
  Shift Arithmetic2 : ArithShift  BitShiftNumber=6  BitShiftDirection=Left
  Shift Arithmetic3 : ArithShift  BitShiftNumber=7  BitShiftDirection=Left
  Shift Arithmetic4 : ArithShift
  Shift Arithmetic5 : ArithShift  BitShiftNumber=1  BitShiftDirection=Left
  Shift Arithmetic6 : ArithShift  BitShiftNumber=2  BitShiftDirection=Left
  Shift Arithmetic7 : ArithShift  BitShiftNumber=3  BitShiftDirection=Left
  Sum : Sum  Inputs=++++++++
  Command Speed : Outport
  wires:
  Digital Input/1 -> Data Type Conversion/1
  Digital Input1/1 -> Data Type Conversion1/1
  Digital Input2/1 -> Data Type Conversion2/1
  Digital Input3/1 -> Data Type Conversion3/1
  Digital Input4/1 -> Data Type Conversion4/1
  Digital Input5/1 -> Data Type Conversion7/1
  Digital Input6/1 -> Data Type Conversion5/1
  Digital Input7/1 -> Data Type Conversion6/1
  Sum/1 -> Data Type Conversion8/1
  Data Type Conversion8/1 -> Command Speed/1
  Data Type Conversion/1 -> Shift Arithmetic4/1
  Data Type Conversion1/1 -> Shift Arithmetic5/1
  Data Type Conversion2/1 -> Shift Arithmetic6/1
  Data Type Conversion3/1 -> Shift Arithmetic7/1
  Data Type Conversion4/1 -> Shift Arithmetic/1
  Data Type Conversion7/1 -> Shift Arithmetic1/1
  Data Type Conversion5/1 -> Shift Arithmetic2/1
  Data Type Conversion6/1 -> Shift Arithmetic3/1
  Shift Arithmetic4/1 -> Sum/1
  Shift Arithmetic5/1 -> Sum/2
  Shift Arithmetic6/1 -> Sum/3
  Shift Arithmetic7/1 -> Sum/4
  Shift Arithmetic/1 -> Sum/5
  Shift Arithmetic1/1 -> Sum/6
  Shift Arithmetic2/1 -> Sum/7
  Shift Arithmetic3/1 -> Sum/8

== system template_Final_Project_MPC5643L/High-Level Design/Outputs/Extract x,y,psi ==
  s,n,psi,us : Inport
  Demux : Demux
  Mux : Mux  Inputs=3
  Terminator : Terminator
  s,n to x,y : Veh_Sim/s,n to x,y  SystemSampleTime=-1
  x,y,psi : Outport
  wires:
  Demux/1 -> s,n to x,y/1
  Demux/2 -> s,n to x,y/2
  s,n,psi,us/1 -> Demux/1
  s,n to x,y/1 -> Mux/1
  s,n to x,y/2 -> Mux/2
  Demux/3 -> Mux/3
  Mux/1 -> x,y,psi/1
  Demux/4 -> Terminator/1

== system template_Final_Project_MPC5643L/High-Level Design/Outputs/Extract x,y,psi (Cars 1 - 6) ==
  s,n,psi,us (Cars 1 - 6) : Inport
  Demux : Demux  Outputs=6
  Extract x,y,psi : Subsystem
  Extract x,y,psi1 : Subsystem
  Extract x,y,psi2 : Subsystem
  Extract x,y,psi3 : Subsystem
  Extract x,y,psi4 : Subsystem
  Extract x,y,psi5 : Subsystem
  Mux : Mux  Inputs=6
  x,y,psi (Cars 1 - 6) : Outport
  wires:
  Demux/1 -> Extract x,y,psi/1(s,n,psi,us)
  Extract x,y,psi/1(x,y,psi) -> Mux/1
  Demux/2 -> Extract x,y,psi1/1(s,n,psi,us)
  Extract x,y,psi1/1(x,y,psi) -> Mux/2
  Demux/3 -> Extract x,y,psi2/1(s,n,psi,us)
  Extract x,y,psi2/1(x,y,psi) -> Mux/3
  Demux/4 -> Extract x,y,psi3/1(s,n,psi,us)
  Extract x,y,psi3/1(x,y,psi) -> Mux/4
  Demux/5 -> Extract x,y,psi4/1(s,n,psi,us)
  Extract x,y,psi4/1(x,y,psi) -> Mux/5
  s,n,psi,us (Cars 1 - 6)/1 -> Demux/1
  Mux/1 -> x,y,psi (Cars 1 - 6)/1
  Extract x,y,psi5/1(x,y,psi) -> Mux/6
  Demux/6 -> Extract x,y,psi5/1(s,n,psi,us)

== system template_Final_Project_MPC5643L/High-Level Design/Outputs/Scale ==
  torque : Inport
  Sum : Sum  Inputs=|++
  offset : Constant  Value=.5  OutDataTypeStr=single
  torque gain : Gain  Gain=3.162*10^-4
  duty cycle : Outport
  wires:
  Sum/1 -> duty cycle/1
  torque gain/1 -> Sum/1
  offset/1 -> Sum/2
  torque/1 -> torque gain/1

== system template_Final_Project_MPC5643L/High-Level Design/Outputs/Tx CAN ==
  s,n,psi,us : Inport
  CAN Transmit : rappid_564xl_ec_toolbox/MPC564xL/Communication Blocks/CAN Transmit  can_unit=A  can_unit_v2=0  can_buffer=0  can_id=45
  CAN Transmit1 : rappid_564xl_ec_toolbox/MPC564xL/Communication Blocks/CAN Transmit  can_unit=A  can_unit_v2=0  can_buffer=1  can_id=46
  Constant : Constant  Value=8  OutDataTypeStr=uint8
  Constant1 : Constant  Value=8  OutDataTypeStr=uint8
  Demux : Demux
  Mux : Mux  Inputs=2
  Mux1 : Mux  Inputs=2
  Single to Bytes{,1..3} (4 alike) : Conv_Lib/Single to Bytes
  wires:
  Constant1/1 -> CAN Transmit1/2
  Single to Bytes/1 -> Mux/1
  Single to Bytes1/1 -> Mux/2
  Single to Bytes2/1 -> Mux1/1
  Single to Bytes3/1 -> Mux1/2
  Mux/1 -> CAN Transmit/1
  Demux/1 -> Single to Bytes/1
  Demux/2 -> Single to Bytes1/1
  Demux/3 -> Single to Bytes3/1
  Demux/4 -> Single to Bytes2/1
  s,n,psi,us/1 -> Demux/1
  Constant/1 -> CAN Transmit/2
  Mux1/1 -> CAN Transmit1/1

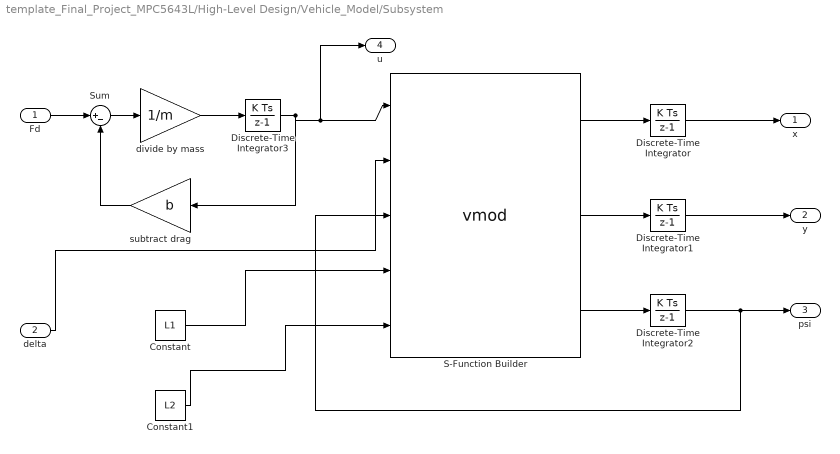
== system template_Final_Project_MPC5643L/High-Level Design/Vehicle_Model/Subsystem ==
  Fd : Inport
  delta : Inport  Port=2
  Constant : Constant  Value=L1  OutDataTypeStr=single
  Constant1 : Constant  Value=L2  OutDataTypeStr=single
  Discrete-Time Integrator{,1..3} (4 alike) : DiscreteIntegrator  SampleTime=-1  ICPrevOutput=DiscIntNeverNeededParam  ICPrevScaledInput=DiscIntNeverNeededParam
  S-Function Builder : S-Function  InitFcn=try, set_param(gcb,'FunctionName','vmod'), end  FunctionName=vmod  SFunctionModules=vmod_wrapper  WizardData=DataTag1  EnableBusSupport=off  mask(S-Function Builder){}
      mask help: Simulink:masks:SFunctionBuilder_MD
      mask init:
      | val = [[.9  0.75 0.75 1 1 .9 .9 1]',[1 1 0.75 0.75 .9 .9 1 .9]'];try , sys = get_param(gcb,'SfunBuilderFcnName');if isempty(sys), sys = get_param(gcb,'FunctionName'); end,catch, sys = get_param(gcb,'FunctionName'); end
      settings: CopyFcn=set_param(gcbh,'LinkStatus','none')  PreSaveFcn=try, set_param(gcb,'FunctionName','vmod'), end  OpenFcn=sfunctionwizard(gcbh)
      mask Display: plot(val(:,1),val(:,2)),disp(sys), port_label('input',1,'u'), port_label('input',2,'delta'), port_label('input',3,'psi'), port_label('input',4,'L1'), port_label('input',5,'L2'), port_label('output',1,'xdot'), port_label('output',2,'ydot'), port_label('output',3,'psidot')
  Sum : Sum  Inputs=|+-
  divide by mass : Gain  Gain=1/m
  subtract drag : Gain  Gain=b
  x : Outport
  y : Outport  Port=2
  psi : Outport  Port=3
  u : Outport  Port=4
  wires:
  delta/1 -> S-Function Builder/2
  S-Function Builder/1 -> Discrete-Time Integrator/1
  S-Function Builder/2 -> Discrete-Time Integrator1/1
  S-Function Builder/3 -> Discrete-Time Integrator2/1
  Discrete-Time Integrator/1 -> x/1
  Discrete-Time Integrator1/1 -> y/1
  Discrete-Time Integrator2/1 -> psi/1, S-Function Builder/3
  Fd/1 -> Sum/1
  Sum/1 -> divide by mass/1
  divide by mass/1 -> Discrete-Time Integrator3/1
  Discrete-Time Integrator3/1 -> subtract drag/1, S-Function Builder/1, u/1
  subtract drag/1 -> Sum/2
  Constant/1 -> S-Function Builder/4
  Constant1/1 -> S-Function Builder/5

== system template_Final_Project_MPC5643L/High-Level Design/Vehicle_Model/u to us ==
  s : Inport
  psi : Inport  Port=2
  delta : Inport  Port=3
  u : Inport  Port=4
  Look up the Forward Vector : Veh_Sim/x,y to s,n/Look up the Forward Vector  SystemSampleTime=-1
  Product : Product  RndMeth=Zero
  Product1 : Product  RndMeth=Zero
  Product2 : Product  RndMeth=Zero
  Sum : Sum  Inputs=+|+
  Sum1 : Sum  Inputs=|++
  Trigonometric Function : Trigonometry  Operator=cos
  Trigonometric Function1 : Trigonometry
  us : Outport
  wires:
  s/1 -> Look up the Forward Vector/1
  psi/1 -> Sum/1
  delta/1 -> Sum/2
  Sum/1 -> Trigonometric Function1/1, Trigonometric Function/1
  Look up the Forward Vector/1 -> Product1/1
  Trigonometric Function/1 -> Product1/2
  Look up the Forward Vector/2 -> Product/1
  Trigonometric Function1/1 -> Product/2
  Product/1 -> Sum1/1
  Product1/1 -> Sum1/2
  Sum1/1 -> Product2/1
  u/1 -> Product2/2
  Product2/1 -> us/1

== system template_Final_Project_MPC5643L/High-Level Design/ACC/ACC State Logic/Pick_Lead ==
  H : Inport
  si : Inport  Port=2
  s : Inport  Port=3
  S-Function Builder : S-Function  InitFcn=try, set_param(gcb,'FunctionName','PL'), end  FunctionName=PL  SFunctionModules=PL_wrapper  WizardData=DataTag0  EnableBusSupport=off  mask(S-Function Builder){}
      mask help: Simulink:masks:SFunctionBuilder_MD
      mask init: same as template_Final_Project_MPC5643L/High-Level Design/Vehicle_Model/Subsystem/S-Function Builder
      settings: CopyFcn=set_param(gcbh,'LinkStatus','none')  PreSaveFcn=try, set_param(gcb,'FunctionName','PL'), end  OpenFcn=sfunctionwizard(gcbh)
      mask Display: plot(val(:,1),val(:,2)),disp(sys), port_label('input',1,'H'), port_label('input',2,'si'), port_label('input',3,'s'), port_label('output',1,'lead_s'), port_label('output',2,'lead_u')
  lead_s : Outport
  lead_u : Outport  Port=2
  wires:
  S-Function Builder/1 -> lead_s/1
  S-Function Builder/2 -> lead_u/1
  H/1 -> S-Function Builder/1
  si/1 -> S-Function Builder/2
  s/1 -> S-Function Builder/3

== system template_Final_Project_MPC5643L/High-Level Design/ACC/Speed Ctrl/PI ==
  Error : Inport
  Gain : Gain  Gain=V_Ki  SaturateOnIntegerOverflow=on  OutDataTypeStr=Inherit: Same as input  ParamDataTypeStr=Inherit: Same as input
  Gain1 : Gain  Gain=V_Kp  SaturateOnIntegerOverflow=on  OutDataTypeStr=Inherit: Same as input  ParamDataTypeStr=Inherit: Same as input
  My Discrete Integrator : Subsystem
  Sum : Sum  Inputs=|++  SaturateOnIntegerOverflow=on
  U : Outport
  wires:
  Gain/1 -> My Discrete Integrator/1(X_dot)
  My Discrete Integrator/1(X) -> Sum/1
  Gain1/1 -> Sum/2
  Error/1 -> Gain/1, Gain1/1
  Sum/1 -> U/1

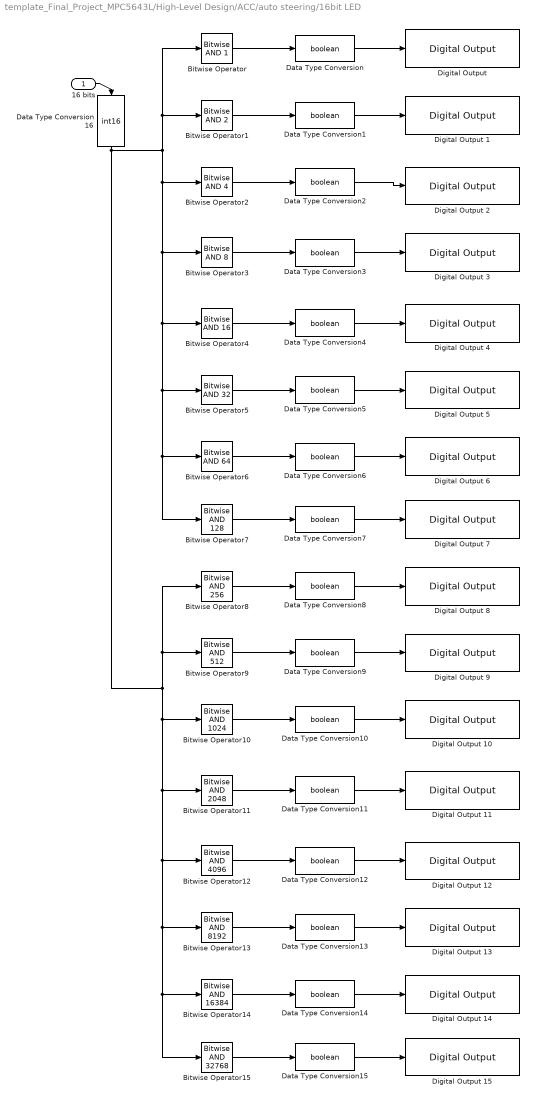
== system template_Final_Project_MPC5643L/High-Level Design/ACC/auto steering/16bit LED ==
  16 bits : Inport
  Bitwise Operator : simulink/Logic and Bit Operations/Bitwise Operator  logicop=AND  UseBitMask=on  BitMask=1  BitMaskRealWorld=Stored Integer
  Bitwise Operator1 : simulink/Logic and Bit Operations/Bitwise Operator  logicop=AND  UseBitMask=on  BitMask=2  BitMaskRealWorld=Stored Integer
  Bitwise Operator10 : simulink/Logic and Bit Operations/Bitwise Operator  logicop=AND  UseBitMask=on  BitMask=1024  BitMaskRealWorld=Stored Integer
  Bitwise Operator11 : simulink/Logic and Bit Operations/Bitwise Operator  logicop=AND  UseBitMask=on  BitMask=2048  BitMaskRealWorld=Stored Integer
  Bitwise Operator12 : simulink/Logic and Bit Operations/Bitwise Operator  logicop=AND  UseBitMask=on  BitMask=4096  BitMaskRealWorld=Stored Integer
  Bitwise Operator13 : simulink/Logic and Bit Operations/Bitwise Operator  logicop=AND  UseBitMask=on  BitMask=8192  BitMaskRealWorld=Stored Integer
  Bitwise Operator14 : simulink/Logic and Bit Operations/Bitwise Operator  logicop=AND  UseBitMask=on  BitMask=16384  BitMaskRealWorld=Stored Integer
  Bitwise Operator15 : simulink/Logic and Bit Operations/Bitwise Operator  logicop=AND  UseBitMask=on  BitMask=32768  BitMaskRealWorld=Stored Integer
  Bitwise Operator2 : simulink/Logic and Bit Operations/Bitwise Operator  logicop=AND  UseBitMask=on  BitMask=4  BitMaskRealWorld=Stored Integer
  Bitwise Operator3 : simulink/Logic and Bit Operations/Bitwise Operator  logicop=AND  UseBitMask=on  BitMask=8  BitMaskRealWorld=Stored Integer
  Bitwise Operator4 : simulink/Logic and Bit Operations/Bitwise Operator  logicop=AND  UseBitMask=on  BitMask=16  BitMaskRealWorld=Stored Integer
  Bitwise Operator5 : simulink/Logic and Bit Operations/Bitwise Operator  logicop=AND  UseBitMask=on  BitMask=32  BitMaskRealWorld=Stored Integer
  Bitwise Operator6 : simulink/Logic and Bit Operations/Bitwise Operator  logicop=AND  UseBitMask=on  BitMask=64  BitMaskRealWorld=Stored Integer
  Bitwise Operator7 : simulink/Logic and Bit Operations/Bitwise Operator  logicop=AND  UseBitMask=on  BitMask=128  BitMaskRealWorld=Stored Integer
  Bitwise Operator8 : simulink/Logic and Bit Operations/Bitwise Operator  logicop=AND  UseBitMask=on  BitMask=256  BitMaskRealWorld=Stored Integer
  Bitwise Operator9 : simulink/Logic and Bit Operations/Bitwise Operator  logicop=AND  UseBitMask=on  BitMask=512  BitMaskRealWorld=Stored Integer
  Data Type Conversion{,1..15} (16 alike) : DataTypeConversion  OutDataTypeStr=boolean
  Data Type Conversion16 : DataTypeConversion  OutDataTypeStr=int16
  "Digital Output " : rappid_564xl_ec_toolbox/MPC564xL/General Purpose Blocks/Digital Output   gpio_outputs="43  : PC11 : [ 80 ] : [ M14 ]"  pinNum=[ 80 ]  pcrNum=43
  Digital Output 1 : rappid_564xl_ec_toolbox/MPC564xL/General Purpose Blocks/Digital Output   gpio_outputs="44  : PC12 : [ 82 ] : [ N15 ]"  pinNum=[ 82 ]  pcrNum=44
  Digital Output 10 : rappid_564xl_ec_toolbox/MPC564xL/General Purpose Blocks/Digital Output   gpio_outputs="53  : PD5  : [ 33 ] : [ N3 ]"  pinNum=[ 33 ]  pcrNum=53
  Digital Output 11 : rappid_564xl_ec_toolbox/MPC564xL/General Purpose Blocks/Digital Output   gpio_outputs="54  : PD6  : [ 34 ] : [ P3 ]"  pinNum=[ 34 ]  pcrNum=54
  Digital Output 12 : rappid_564xl_ec_toolbox/MPC564xL/General Purpose Blocks/Digital Output   gpio_outputs="55  : PD7  : [ 37 ] : [ R4 ]"  pinNum=[ 37 ]  pcrNum=55
  Digital Output 13 : rappid_564xl_ec_toolbox/MPC564xL/General Purpose Blocks/Digital Output   gpio_outputs="56  : PD8  : [ 32 ] : [ M3 ]"  pinNum=[ 32 ]  pcrNum=56
  Digital Output 14 : rappid_564xl_ec_toolbox/MPC564xL/General Purpose Blocks/Digital Output   gpio_outputs="57  : PD9  : [ 26 ] : [ L3 ]"  pinNum=[ 26 ]  pcrNum=57
  Digital Output 15 : rappid_564xl_ec_toolbox/MPC564xL/General Purpose Blocks/Digital Output   gpio_outputs="58  : PD10 : [ 76 ] : [ T15 ]"  pinNum=[ 76 ]  pcrNum=58
  Digital Output 2 : rappid_564xl_ec_toolbox/MPC564xL/General Purpose Blocks/Digital Output   gpio_outputs="45  : PC13 : [ 101 ] : [ F15 ]"  pinNum=[ 101 ]  pcrNum=45
  Digital Output 3 : rappid_564xl_ec_toolbox/MPC564xL/General Purpose Blocks/Digital Output   gpio_outputs="46  : PC14 : [ 103 ] : [ E15 ]"  pinNum=[ 103 ]  pcrNum=46
  Digital Output 4 : rappid_564xl_ec_toolbox/MPC564xL/General Purpose Blocks/Digital Output   gpio_outputs="47  : PC15 : [ 124 ] : [ A8 ]"  pinNum=[ 124 ]  pcrNum=47
  Digital Output 5 : rappid_564xl_ec_toolbox/MPC564xL/General Purpose Blocks/Digital Output   gpio_outputs="48  : PD0  : [ 125 ] : [ B8 ]"  pinNum=[ 125 ]  pcrNum=48
  Digital Output 6 : rappid_564xl_ec_toolbox/MPC564xL/General Purpose Blocks/Digital Output   gpio_outputs="49  : PD1  : [ 3 ] : [ E3 ]"  pinNum=[ 3 ]  pcrNum=49
  Digital Output 7 : rappid_564xl_ec_toolbox/MPC564xL/General Purpose Blocks/Digital Output   gpio_outputs="50  : PD2  : [ 140 ] : [ C5 ]"  pinNum=[ 140 ]  pcrNum=50
  Digital Output 8 : rappid_564xl_ec_toolbox/MPC564xL/General Purpose Blocks/Digital Output   gpio_outputs="51  : PD3  : [ 128 ] : [ A7 ]"  pinNum=[ 128 ]  pcrNum=51
  Digital Output 9 : rappid_564xl_ec_toolbox/MPC564xL/General Purpose Blocks/Digital Output   gpio_outputs="52  : PD4  : [ 129 ] : [ B7 ]"  pinNum=[ 129 ]  pcrNum=52
  wires:
  Data Type Conversion16/1 -> Bitwise Operator10/1, Bitwise Operator11/1, Bitwise Operator12/1, Bitwise Operator13/1, Bitwise Operator14/1, Bitwise Operator15/1, Bitwise Operator9/1, Bitwise Operator8/1, Bitwise Operator/1, Bitwise Operator1/1, Bitwise Operator7/1, Bitwise Operator6/1, Bitwise Operator5/1, Bitwise Operator4/1, Bitwise Operator3/1, Bitwise Operator2/1
  Bitwise Operator15/1 -> Data Type Conversion15/1
  Data Type Conversion15/1 -> Digital Output 15/1
  Bitwise Operator14/1 -> Data Type Conversion14/1
  Data Type Conversion14/1 -> Digital Output 14/1
  Bitwise Operator13/1 -> Data Type Conversion13/1
  Data Type Conversion13/1 -> Digital Output 13/1
  Bitwise Operator8/1 -> Data Type Conversion8/1
  Bitwise Operator9/1 -> Data Type Conversion9/1
  Bitwise Operator10/1 -> Data Type Conversion10/1
  Bitwise Operator11/1 -> Data Type Conversion11/1
  Bitwise Operator12/1 -> Data Type Conversion12/1
  Data Type Conversion8/1 -> Digital Output 8/1
  Data Type Conversion9/1 -> Digital Output 9/1
  Data Type Conversion10/1 -> Digital Output 10/1
  Data Type Conversion11/1 -> Digital Output 11/1
  Data Type Conversion12/1 -> Digital Output 12/1
  Bitwise Operator7/1 -> Data Type Conversion7/1
  Data Type Conversion7/1 -> Digital Output 7/1
  Bitwise Operator6/1 -> Data Type Conversion6/1
  Data Type Conversion6/1 -> Digital Output 6/1
  Bitwise Operator5/1 -> Data Type Conversion5/1
  Data Type Conversion5/1 -> Digital Output 5/1
  Bitwise Operator/1 -> Data Type Conversion/1
  Bitwise Operator1/1 -> Data Type Conversion1/1
  Bitwise Operator2/1 -> Data Type Conversion2/1
  Bitwise Operator3/1 -> Data Type Conversion3/1
  Bitwise Operator4/1 -> Data Type Conversion4/1
  16 bits/1 -> Data Type Conversion16/1
  Data Type Conversion/1 -> "Digital Output "/1
  Data Type Conversion1/1 -> Digital Output 1/1
  Data Type Conversion2/1 -> Digital Output 2/1
  Data Type Conversion3/1 -> Digital Output 3/1
  Data Type Conversion4/1 -> Digital Output 4/1

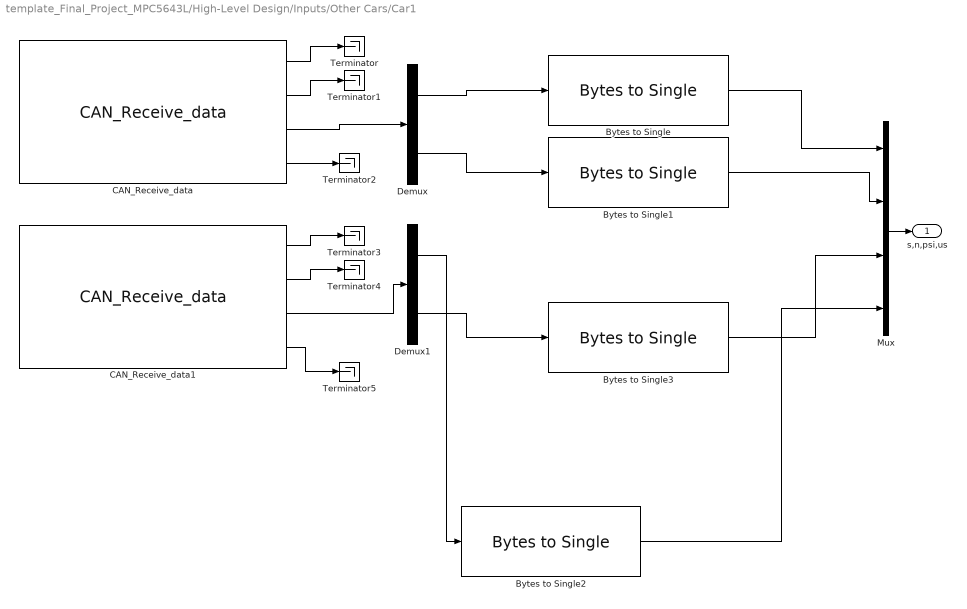
== system template_Final_Project_MPC5643L/High-Level Design/Inputs/Other Cars/Car1 ==
  Bytes to Single{,1..3} (4 alike) : Conv_Lib/Bytes to Single
  CAN_Receive_data : rappid_564xl_ec_toolbox/MPC564xL/Communication Blocks/CAN_Receive_data  can_unit=A  can_unit_v2=0  can_buffer=2  can_id=15
  CAN_Receive_data1 : rappid_564xl_ec_toolbox/MPC564xL/Communication Blocks/CAN_Receive_data  can_unit=A  can_unit_v2=0  can_buffer=3  can_id=16
  Demux : Demux  Outputs=2
  Demux1 : Demux  Outputs=2
  Mux : Mux
  Terminator{,1..5} (6 alike) : Terminator
  s,n,psi,us : Outport
  wires:
  Bytes to Single1/1 -> Mux/2
  Bytes to Single3/1 -> Mux/3
  Demux/1 -> Bytes to Single/1
  Demux/2 -> Bytes to Single1/1
  Demux1/1 -> Bytes to Single2/1
  Demux1/2 -> Bytes to Single3/1
  Bytes to Single/1 -> Mux/1
  Bytes to Single2/1 -> Mux/4
  Mux/1 -> s,n,psi,us/1
  CAN_Receive_data/1 -> Terminator/1
  CAN_Receive_data/2 -> Terminator1/1
  CAN_Receive_data/3 -> Demux/1
  CAN_Receive_data/4 -> Terminator2/1
  CAN_Receive_data1/1 -> Terminator3/1
  CAN_Receive_data1/2 -> Terminator4/1
  CAN_Receive_data1/3 -> Demux1/1
  CAN_Receive_data1/4 -> Terminator5/1

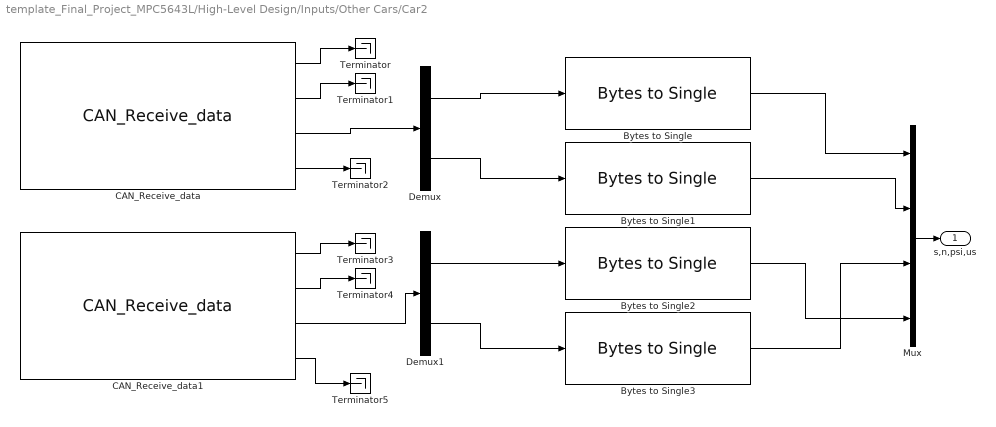
== system template_Final_Project_MPC5643L/High-Level Design/Inputs/Other Cars/Car2 ==
  Bytes to Single{,1..3} (4 alike) : Conv_Lib/Bytes to Single
  CAN_Receive_data : rappid_564xl_ec_toolbox/MPC564xL/Communication Blocks/CAN_Receive_data  can_unit=A  can_unit_v2=0  can_buffer=4  can_id=25
  CAN_Receive_data1 : rappid_564xl_ec_toolbox/MPC564xL/Communication Blocks/CAN_Receive_data  can_unit=A  can_unit_v2=0  can_buffer=5  can_id=26
  Demux : Demux  Outputs=2
  Demux1 : Demux  Outputs=2
  Mux : Mux
  Terminator{,1..5} (6 alike) : Terminator
  s,n,psi,us : Outport
  wires:
  CAN_Receive_data1/4 -> Terminator5/1
  CAN_Receive_data1/3 -> Demux1/1
  CAN_Receive_data1/2 -> Terminator4/1
  CAN_Receive_data1/1 -> Terminator3/1
  CAN_Receive_data/4 -> Terminator2/1
  CAN_Receive_data/3 -> Demux/1
  CAN_Receive_data/2 -> Terminator1/1
  CAN_Receive_data/1 -> Terminator/1
  Mux/1 -> s,n,psi,us/1
  Bytes to Single2/1 -> Mux/4
  Bytes to Single/1 -> Mux/1
  Demux1/2 -> Bytes to Single3/1
  Demux1/1 -> Bytes to Single2/1
  Demux/2 -> Bytes to Single1/1
  Demux/1 -> Bytes to Single/1
  Bytes to Single3/1 -> Mux/3
  Bytes to Single1/1 -> Mux/2

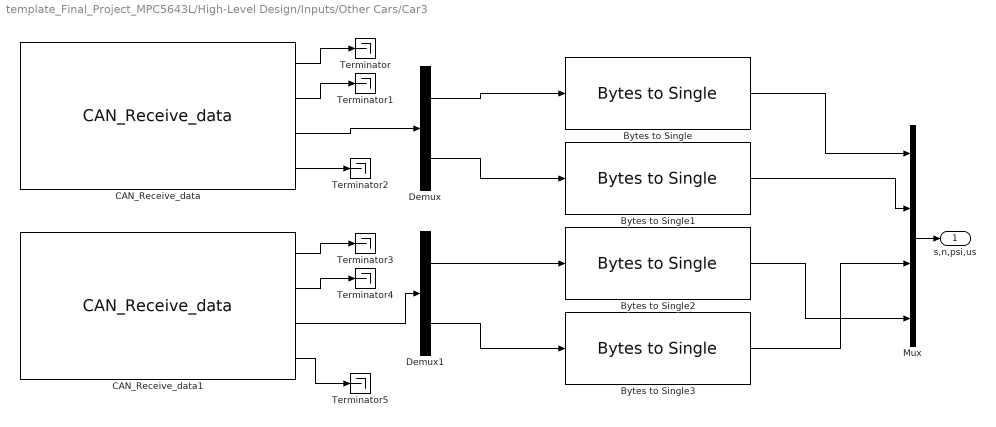
== system template_Final_Project_MPC5643L/High-Level Design/Inputs/Other Cars/Car3 ==
  Bytes to Single{,1..3} (4 alike) : Conv_Lib/Bytes to Single
  CAN_Receive_data : rappid_564xl_ec_toolbox/MPC564xL/Communication Blocks/CAN_Receive_data  can_unit=A  can_unit_v2=0  can_buffer=6  can_id=35
  CAN_Receive_data1 : rappid_564xl_ec_toolbox/MPC564xL/Communication Blocks/CAN_Receive_data  can_unit=A  can_unit_v2=0  can_buffer=7  can_id=36
  Demux : Demux  Outputs=2
  Demux1 : Demux  Outputs=2
  Mux : Mux
  Terminator{,1..5} (6 alike) : Terminator
  s,n,psi,us : Outport
  wires:
  Bytes to Single1/1 -> Mux/2
  Bytes to Single3/1 -> Mux/3
  Demux/1 -> Bytes to Single/1
  Demux/2 -> Bytes to Single1/1
  Demux1/1 -> Bytes to Single2/1
  Demux1/2 -> Bytes to Single3/1
  Bytes to Single/1 -> Mux/1
  Bytes to Single2/1 -> Mux/4
  Mux/1 -> s,n,psi,us/1
  CAN_Receive_data/1 -> Terminator/1
  CAN_Receive_data/2 -> Terminator1/1
  CAN_Receive_data/3 -> Demux/1
  CAN_Receive_data/4 -> Terminator2/1
  CAN_Receive_data1/1 -> Terminator3/1
  CAN_Receive_data1/2 -> Terminator4/1
  CAN_Receive_data1/3 -> Demux1/1
  CAN_Receive_data1/4 -> Terminator5/1

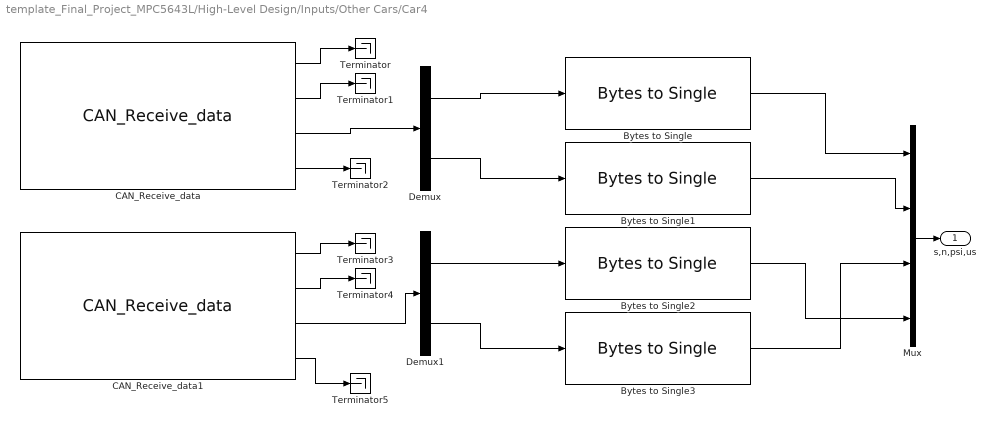
== system template_Final_Project_MPC5643L/High-Level Design/Inputs/Other Cars/Car4 ==
  Bytes to Single{,1..3} (4 alike) : Conv_Lib/Bytes to Single
  CAN_Receive_data : rappid_564xl_ec_toolbox/MPC564xL/Communication Blocks/CAN_Receive_data  can_unit=A  can_unit_v2=0  can_buffer=8  can_id=75
  CAN_Receive_data1 : rappid_564xl_ec_toolbox/MPC564xL/Communication Blocks/CAN_Receive_data  can_unit=A  can_unit_v2=0  can_buffer=9  can_id=76
  Demux : Demux  Outputs=2
  Demux1 : Demux  Outputs=2
  Mux : Mux
  Terminator{,1..5} (6 alike) : Terminator
  s,n,psi,us : Outport
  wires:
  CAN_Receive_data1/4 -> Terminator5/1
  CAN_Receive_data1/3 -> Demux1/1
  CAN_Receive_data1/2 -> Terminator4/1
  CAN_Receive_data1/1 -> Terminator3/1
  CAN_Receive_data/4 -> Terminator2/1
  CAN_Receive_data/3 -> Demux/1
  CAN_Receive_data/2 -> Terminator1/1
  CAN_Receive_data/1 -> Terminator/1
  Mux/1 -> s,n,psi,us/1
  Bytes to Single2/1 -> Mux/4
  Bytes to Single/1 -> Mux/1
  Demux1/2 -> Bytes to Single3/1
  Demux1/1 -> Bytes to Single2/1
  Demux/2 -> Bytes to Single1/1
  Demux/1 -> Bytes to Single/1
  Bytes to Single3/1 -> Mux/3
  Bytes to Single1/1 -> Mux/2
